simulink model "CSTR"  (R2021a)
settings: Solver=VariableStepAuto  StartTime=0.0  StopTime=999  RelTol=1e-3
undefined symbols (not defined in the file or in its folder): Cp, Cvalve, d, dH, Ea, ko, R, rho
settings Model: Creator=kpowell  LastModifiedBy=ethan
settings SolverCC: AlgebraicLoopSolver=TrustRegion
settings DataIOCC: ReturnWorkspaceOutputs=off
settings DebuggingCC: SFMachineParentedDataDiag=warning  ArithmeticOperatorsInVariantConditions=warning
settings SFSimCC: CustomCodeUndefinedFunction=UseInterfaceOnly

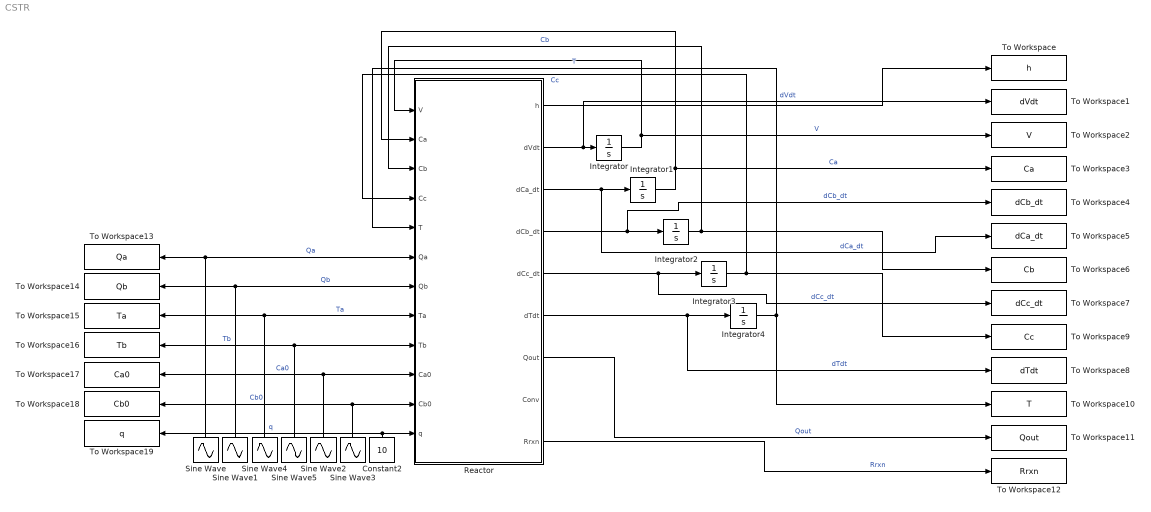
== system CSTR ==
  Constant2 : Constant  Value=10
  Integrator : Integrator  InitialCondition=70
  Integrator1 : Integrator  InitialCondition=5
  Integrator2 : Integrator  InitialCondition=5
  Integrator3 : Integrator
  Integrator4 : Integrator  InitialCondition=500
  Reactor : MATLAB Function  TreatAsAtomicUnit=on
  Sine Wave : Sin  Amplitude=4  Bias=5  Frequency=.01  SampleTime=0.1
  Sine Wave1 : Sin  Amplitude=4  Bias=5  Frequency=.01  Phase=1.5707963267948966192313216916398  SampleTime=0.01
  Sine Wave2 : Sin  Amplitude=10  Bias=15  Frequency=.1  Phase=1.5707963267948966192313216916398  SampleTime=0.1
  Sine Wave3 : Sin  Amplitude=10  Bias=15  Frequency=.08  SampleTime=0.1
  Sine Wave4 : Sin  Amplitude=50  Bias=400  Frequency=.05  SampleTime=0.1
  Sine Wave5 : Sin  Amplitude=50  Bias=400  Frequency=.05  Phase=1.5  SampleTime=0.1
  To Workspace : ToWorkspace  VariableName=h  SampleTime=1
  To Workspace1 : ToWorkspace  VariableName=dVdt  SampleTime=1
  To Workspace10 : ToWorkspace  VariableName=T  SampleTime=1
  To Workspace11 : ToWorkspace  VariableName=Qout  SampleTime=1
  To Workspace12 : ToWorkspace  VariableName=Rrxn  SampleTime=1
  To Workspace13 : ToWorkspace  VariableName=Qa  SampleTime=1
  To Workspace14 : ToWorkspace  VariableName=Qb  SampleTime=1
  To Workspace15 : ToWorkspace  VariableName=Ta  SampleTime=1
  To Workspace16 : ToWorkspace  VariableName=Tb  SampleTime=1
  To Workspace17 : ToWorkspace  VariableName=Ca0  SampleTime=1
  To Workspace18 : ToWorkspace  VariableName=Cb0  SampleTime=1
  To Workspace19 : ToWorkspace  VariableName=q  SampleTime=1
  To Workspace2 : ToWorkspace  VariableName=V  SampleTime=1
  To Workspace3 : ToWorkspace  VariableName=Ca  SampleTime=1
  To Workspace4 : ToWorkspace  VariableName=dCb_dt  SampleTime=1
  To Workspace5 : ToWorkspace  VariableName=dCa_dt  SampleTime=1
  To Workspace6 : ToWorkspace  VariableName=Cb  SampleTime=1
  To Workspace7 : ToWorkspace  VariableName=dCc_dt  SampleTime=1
  To Workspace8 : ToWorkspace  VariableName=dTdt  SampleTime=1
  To Workspace9 : ToWorkspace  VariableName=Cc  SampleTime=1
  wires:
  Reactor/6(dTdt) -> To Workspace8/1, Integrator4/1  "dTdt"
  Reactor/5(dCc_dt) -> To Workspace7/1, Integrator3/1  "dCc_dt"
  Reactor/4(dCb_dt) -> To Workspace4/1, Integrator2/1  "dCb_dt"
  Reactor/3(dCa_dt) -> To Workspace5/1, Integrator1/1  "dCa_dt"
  Reactor/2(dVdt) -> To Workspace1/1, Integrator/1  "dVdt"
  Integrator/1 -> To Workspace2/1, Reactor/1(V)  "V"
  Integrator1/1 -> To Workspace3/1, Reactor/2(Ca)  "Ca"
  Integrator2/1 -> To Workspace6/1, Reactor/3(Cb)  "Cb"
  Integrator3/1 -> To Workspace9/1, Reactor/4(Cc)  "Cc"
  Integrator4/1 -> To Workspace10/1, Reactor/5(T)  "T"
  Sine Wave/1 -> To Workspace13/1, Reactor/6(Qa)  "Qa"
  Sine Wave1/1 -> To Workspace14/1, Reactor/7(Qb)  "Qb"
  Sine Wave4/1 -> To Workspace15/1, Reactor/8(Ta)  "Ta"
  Sine Wave5/1 -> To Workspace16/1, Reactor/9(Tb)  "Tb"
  Sine Wave2/1 -> To Workspace17/1, Reactor/10(Ca0)  "Ca0"
  Sine Wave3/1 -> To Workspace18/1, Reactor/11(Cb0)  "Cb0"
  Constant2/1 -> To Workspace19/1, Reactor/12(q)  "q"
  Reactor/7(Qout) -> To Workspace11/1  "Qout"
  Reactor/9(Rrxn) -> To Workspace12/1  "Rrxn"
  Reactor/1(h) -> To Workspace/1

== matlab function CSTR/Reactor ==
  data: h output; V input; dVdt output; Ca input; Cb input; Cc input; T input; Qa input; Qb input; Ta input; Tb input; Ca0 input; Cb0 input; q input; dCa_dt output; dCb_dt output; dCc_dt output; dTdt output; Qout output; d parameter; Cvalve parameter; dH parameter; Ea parameter; ko parameter; R parameter; Cp parameter; rho parameter; Conv output; Rrxn output
function [h,dVdt,dCa_dt,dCb_dt,dCc_dt,dTdt,Qout,Conv, Rrxn] = reactor(V, Ca, Cb,...
    Cc,T, Qa, Qb, Ta, Tb, Ca0, Cb0, q, d, Cvalve, dH, Ea, ko, R, Cp, rho)

h = V/(pi*d^2/4); %m, height of fluid in tank

Qout = Cvalve*sqrt(h); %m^3, quantity out

Rrxn = ko*exp(-Ea/(R*T))*Ca*Cb*V; %kmol/min, reaction rate

dVdt = Qa+Qb-Qout; %m^3/s change in volume
dCa_dt = (Qa*Ca0-Rrxn-Qout*Ca-Ca*dVdt)/V; %(kmol/m^3)/s, change in [A]
dCb_dt = (Qb*Cb0-Rrxn-Qout*Cb-Cb*dVdt)/V; %(kmol/m^3)/s, change in [B]
dCc_dt = (Rrxn-Qout*Cc-Cc*dVdt)/V; %(kmol/m^3)/s, change in [C]

q = q*1e6; %kJ, incoming heat

dTdt = ((Qa*rho*Cp*Ta+Qb*rho*Cp*Tb-Qout*rho*Cp*T-...
    Rrxn*dH+q)/(rho*Cp)-T*dVdt)/V; %K/s change in temperature

Conv = (Qa*Ca0-Qout*Ca)/(Qa*Ca0); % Conversion rate
